simulink model "Shravan_APS_LQR"  (R2019a)
settings: Solver=VariableStepAuto  StartTime=0.0  StopTime=20  RelTol=1e-3
libraries: Solver_SF x1
settings Model: Creator=srai25  LastModifiedBy=srai25

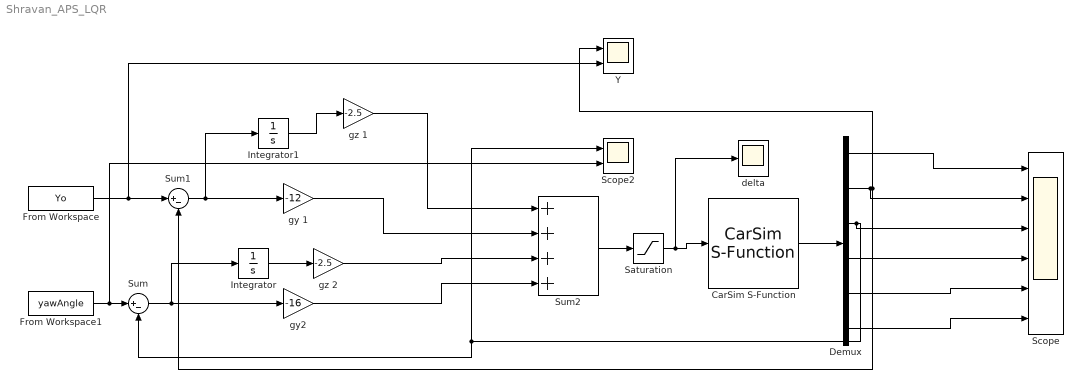
== system Shravan_APS_LQR ==
  CarSim S-Function : Solver_SF/CarSim S-Function  Priority=1  SIMFILE=simfile.sim
  Demux : Demux  Outputs=6
  From Workspace : FromWorkspace  VariableName=Yo  SampleTime=0
  From Workspace1 : FromWorkspace  VariableName=yawAngle  SampleTime=0
  Integrator : Integrator
  Integrator1 : Integrator
  Saturation : Saturate  UpperLimit=280  LowerLimit=-280
  Scope : Scope  NumInputPorts=6
  Scope2 : Scope  NumInputPorts=2
  Sum : Sum  Inputs=|+-
  Sum1 : Sum  Inputs=|+-
  Sum2 : Sum  Inputs=++++
  Y : Scope  NumInputPorts=2
  delta : Scope
  gy 1 : Gain  Gain=-12
  gy2 : Gain  Gain=-16
  gz 1 : Gain  Gain=-2.5
  gz 2 : Gain  Gain=-2.5
  wires:
  Sum/1 -> Integrator/1, gy2/1
  Integrator/1 -> gz 2/1
  Integrator1/1 -> gz 1/1
  Sum1/1 -> Integrator1/1, gy 1/1
  gz 1/1 -> Sum2/1
  gy 1/1 -> Sum2/2
  gz 2/1 -> Sum2/3
  gy2/1 -> Sum2/4
  CarSim S-Function/1 -> Demux/1
  Demux/2 -> Scope/2, Sum1/2, Y/1
  Demux/3 -> Scope/3, Sum/2, Scope2/1
  Demux/1 -> Scope/1
  Demux/4 -> Scope/4
  Demux/5 -> Scope/5
  Demux/6 -> Scope/6
  From Workspace/1 -> Y/2, Sum1/1
  From Workspace1/1 -> Scope2/2, Sum/1
  Sum2/1 -> Saturation/1
  Saturation/1 -> delta/1, CarSim S-Function/1
